simulink model "agc_log2"  (R2017a)
settings: Solver=VariableStepAuto  StartTime=0.0  StopTime=10.0  RelTol=1e-3
libraries: powerlib_meascontrol x1
settings Model: Creator=Jon  LastModifiedBy=Jon

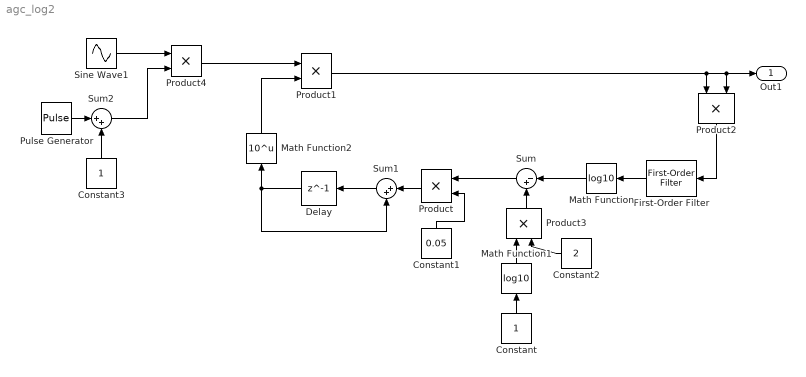
== system agc_log2 ==
  Constant : Constant  SampleTime=6.25e-8
  Constant1 : Constant  Value=0.05  SampleTime=6.25e-8
  Constant2 : Constant  Value=2  SampleTime=6.25e-8
  Constant3 : Constant
  Delay : Delay  DelayLength=1
  First-Order Filter : powerlib_meascontrol/Filters/First-Order Filter  FilterType=Lowpass  Tc=1.09e-6  Ts=6.25e-8  Initialize=on  Vac_Init=[0, 0, 60]  Vdc_Init=0  PlotResponse=off  FreqRange="[0,  200,  1]"
      settings: SourceProductName=Simscape Power Systems
  Math Function : Math  Operator=log10  SaturateOnIntegerOverflow=on
  Math Function1 : Math  Operator=log10  SaturateOnIntegerOverflow=on
  Math Function2 : Math  Operator=10^u  SaturateOnIntegerOverflow=on
  Product{,1..4} (5 alike) : Product
  Pulse Generator : DiscretePulseGenerator  PulseType=Time based  Amplitude=10  Period=0.00003  PulseWidth=50
  Sine Wave1 : Sin  Amplitude=0.1  Frequency=15.7e6  Phase=1  SampleTime=6.25e-8
  Sum : Sum  Inputs=|-+
  Sum1 : Sum  Inputs=|++
  Sum2 : Sum  Inputs=|++
  Out1 : Outport
  wires:
  Product1/1 -> Out1/1, Product2/2, Product2/1
  Product/1 -> Sum1/1
  Delay/1 -> Sum1/2, Math Function2/1
  Math Function2/1 -> Product1/2
  Constant1/1 -> Product/2
  First-Order Filter/1 -> Math Function/1
  Constant/1 -> Math Function1/1
  Product2/1 -> First-Order Filter/1
  Sum/1 -> Product/1
  Sum2/1 -> Product4/2
  Pulse Generator/1 -> Sum2/1
  Sum1/1 -> Delay/1
  Constant2/1 -> Product3/2
  Math Function/1 -> Sum/1
  Constant3/1 -> Sum2/2
  Product3/1 -> Sum/2
  Product4/1 -> Product1/1
  Sine Wave1/1 -> Product4/1
  Math Function1/1 -> Product3/1
